simulink model "model_quad_linear_mpc_est"  (R2021b)
settings: Solver=FixedStepAuto  StartTime=0.0  StopTime=30  FixedStep=.025  RelTol=1e-3
values from neighbouring files (symbols this model uses):
  A = reshape([mt1,mt2,mt3,mt4,mt5,mt6,mt7,mt8],12,12)    [Jacob.m]    (also in Lineared_SS_model.m = reshape([-1.097500e-06;0.000000e+00;0.000000e+00;-4.432200e-; find_optimal_lqr.m = reshape([-1.097500e-06;0.000000e+00;0.000000e+00;-4.432200e-; start_drone.m = zeros(12))
  B = reshape([mt9,mt10],12,4)    [Jacob.m]    (also in Lineared_SS_model.m = reshape([0.000000e+00;0.000000e+00;0.000000e+00;0.000000e+00; find_optimal_lqr.m = reshape([0.000000e+00;0.000000e+00;0.000000e+00;0.000000e+00; nlStateFcn.m = [0 0 0]; start_drone.m = zeros(12,4))
libraries: mpclib x6
settings Model: Creator=Elena  LastModifiedBy=Elena

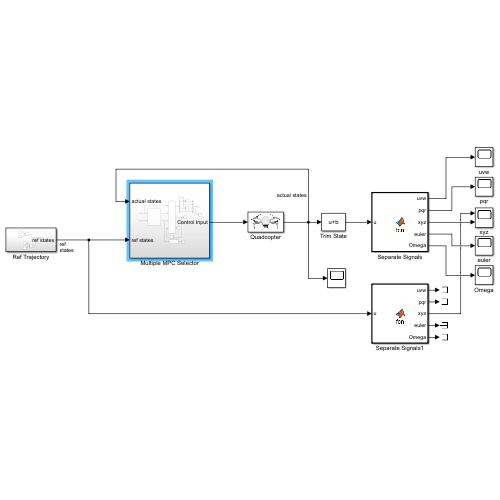
[thumbnail: Simulink's stored preview of the top-level diagram]
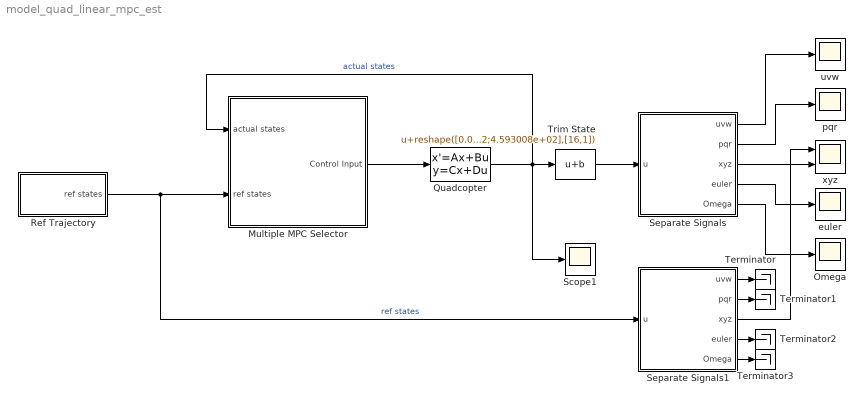
== system model_quad_linear_mpc_est ==
  Multiple MPC Selector : Subsystem
  Omega : Scope
  Quadcopter : StateSpace  A=A  B=B  C=eye(16)  D=zeros(16,4)  InitialCondition=0
      mask Display: image('drone_model.png'); % Use "Edit Image" on toolstrip to change.
  Ref Trajectory : Subsystem
  Scope1 : Scope
  Separate Signals : MATLAB Function  TreatAsAtomicUnit=on
  Separate Signals1 : MATLAB Function  TreatAsAtomicUnit=on
  Terminator{,1..3} (4 alike) : Terminator
  Trim State : Bias  Bias=reshape([0.000000e+00;0.000000e+00;0.000000e+00;0.000000e+00;0.000000e+00;0.000000e+00;0.000000e+00;0.000000e+00;0.000000e+00;0.000000e+00;0.000000e+00;0.000000e+00;0;4.593008e+02;4.593008e+02;4.593008e+02],[16,1])
  euler : Scope
  pqr : Scope
  uvw : Scope
  xyz : Scope  NumInputPorts=2
  wires:
  Quadcopter/1 -> Multiple MPC Selector/1(actual states), Trim State/1, Scope1/1  "actual states"
  Separate Signals/3(xyz) -> xyz/2
  Separate Signals/2(pqr) -> pqr/1
  Separate Signals/1(uvw) -> uvw/1
  Separate Signals/4(euler) -> euler/1
  Separate Signals/5(Omega) -> Omega/1
  Trim State/1 -> Separate Signals/1(u)
  Separate Signals1/3(xyz) -> xyz/1
  Separate Signals1/1(uvw) -> Terminator/1
  Separate Signals1/2(pqr) -> Terminator1/1
  Separate Signals1/4(euler) -> Terminator2/1
  Separate Signals1/5(Omega) -> Terminator3/1
  Ref Trajectory/1(ref states) -> Separate Signals1/1(u), Multiple MPC Selector/2(ref states)  "ref states"
  Multiple MPC Selector/1(Control Input) -> Quadcopter/1

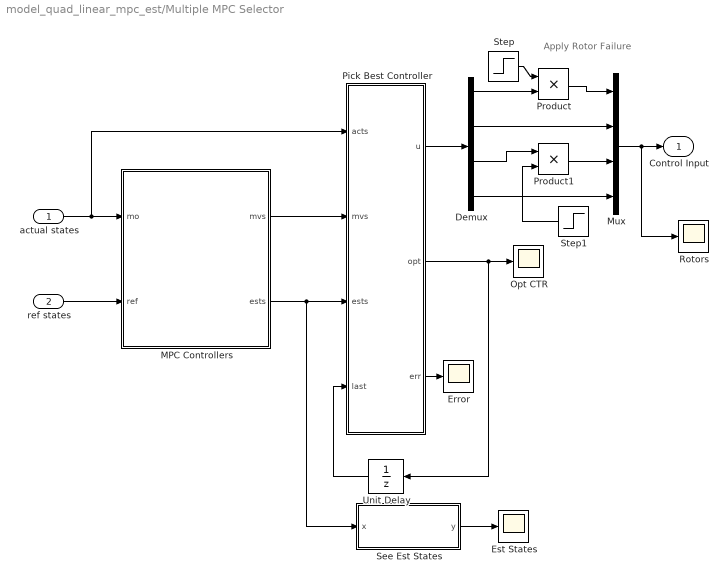
== system model_quad_linear_mpc_est/Multiple MPC Selector ==
  note: Apply Rotor Failure
  actual states : Inport
  ref states : Inport  Port=2
  Demux : Demux
  Error : Scope
  Est States : Scope
  MPC Controllers : Subsystem
  Mux : Mux
  Opt CTR : Scope
  Pick Best Controller : MATLAB Function  TreatAsAtomicUnit=on
  Product : Product
  Product1 : Product
  Rotors : Scope
  See Est States : MATLAB Function  TreatAsAtomicUnit=on
  Step : Step  Time=11  Before=1  After=0  SampleTime=0
  Step1 : Step  Time=21  Before=1  After=0  SampleTime=0
  Unit Delay : UnitDelay  SampleTime=-1  HasFrameUpgradeWarning=on
  Control Input : Outport
  wires:
  actual states/1 -> MPC Controllers/1(mo), Pick Best Controller/1(acts)
  Pick Best Controller/2(opt) -> Opt CTR/1, Unit Delay/1
  Pick Best Controller/3(err) -> Error/1
  Unit Delay/1 -> Pick Best Controller/4(last)
  ref states/1 -> MPC Controllers/2(ref)
  MPC Controllers/1(mvs) -> Pick Best Controller/2(mvs)
  MPC Controllers/2(ests) -> See Est States/1(x), Pick Best Controller/3(ests)
  Demux/2 -> Mux/2
  Step/1 -> Product/1
  Product/1 -> Mux/1
  Mux/1 -> Rotors/1, Control Input/1
  Demux/3 -> Product1/1
  Pick Best Controller/1(u) -> Demux/1
  Demux/1 -> Product/2
  Demux/4 -> Mux/4
  See Est States/1(y) -> Est States/1
  Product1/1 -> Mux/3
  Step1/1 -> Product1/2

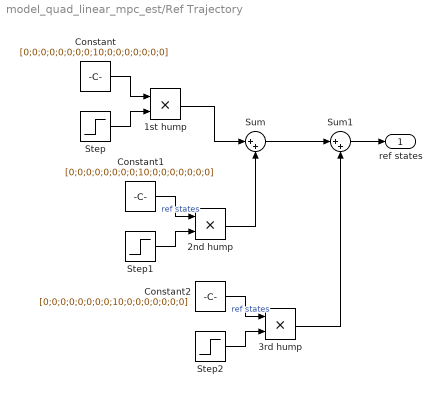
== system model_quad_linear_mpc_est/Ref Trajectory ==
  1st hump : Product
  2nd hump : Product
  3rd hump : Product
  Constant : Constant  Value=[0;0;0;0;0;0;0;0;10;0;0;0;0;0;0;0]
  Constant1 : Constant  Value=[0;0;0;0;0;0;0;0;10;0;0;0;0;0;0;0]
  Constant2 : Constant  Value=[0;0;0;0;0;0;0;0;10;0;0;0;0;0;0;0]
  Step : Step  SampleTime=0
  Step1 : Step  Time=10  SampleTime=0
  Step2 : Step  Time=20  SampleTime=0
  Sum : Sum  Inputs=|++
  Sum1 : Sum  Inputs=|++
  ref states : Outport
  wires:
  Step/1 -> 1st hump/2
  Constant/1 -> 1st hump/1
  Sum1/1 -> ref states/1
  2nd hump/1 -> Sum/2
  Constant1/1 -> 2nd hump/1  "ref states"
  Step1/1 -> 2nd hump/2
  1st hump/1 -> Sum/1
  Constant2/1 -> 3rd hump/1  "ref states"
  3rd hump/1 -> Sum1/2
  Step2/1 -> 3rd hump/2
  Sum/1 -> Sum1/1

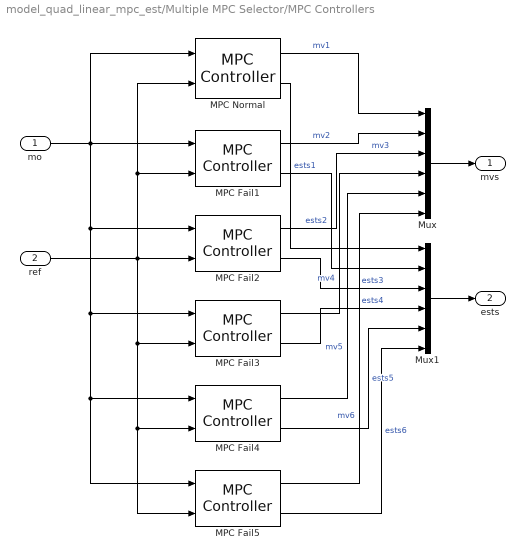
== system model_quad_linear_mpc_est/Multiple MPC Selector/MPC Controllers ==
  mo : Inport
  ref : Inport  Port=2
  MPC Fail1 : mpclib/MPC Controller  SCDEnableBlockLinearizationSpecification=on  mpcobj=mpc_l_fail_1  is_multiple=0  enable_value=0  return_u0=off  updateMPCinCallerWorkspace=on  md_inport=off  mv_inport=off  uref_inport=off  return_cost=off  return_mvseq=off  return_qpstatus=off  return_xseq=off  return_state=on  return_ovseq=off  state_inport=off  umin_inport=off  umax_inport=off  ymin_inport=off  ymax_inport=off  cc_inport=off  ywt_inport=off  uwt_inport=off  duwt_inport=off  rhoeps_inport=off  pm_inport=off  MaximumP=10  HorizonChoice=FixedHorizon  n_ts=0.1  n_p=20  n_mv=4  n_md=0  n_ud=0  n_mo=16  n_uo=0  BlockDataType=double  SampleTimeInherited=off  switch_inport=off
  MPC Fail2 : mpclib/MPC Controller  SCDEnableBlockLinearizationSpecification=on  mpcobj=mpc_l_fail_2  is_multiple=0  enable_value=0  return_u0=off  updateMPCinCallerWorkspace=on  md_inport=off  mv_inport=off  uref_inport=off  return_cost=off  return_mvseq=off  return_qpstatus=off  return_xseq=off  return_state=on  return_ovseq=off  state_inport=off  umin_inport=off  umax_inport=off  ymin_inport=off  ymax_inport=off  cc_inport=off  ywt_inport=off  uwt_inport=off  duwt_inport=off  rhoeps_inport=off  pm_inport=off  MaximumP=10  HorizonChoice=FixedHorizon  n_ts=0.1  n_p=20  n_mv=4  n_md=0  n_ud=0  n_mo=16  n_uo=0  BlockDataType=double  SampleTimeInherited=off  switch_inport=off
  MPC Fail3 : mpclib/MPC Controller  SCDEnableBlockLinearizationSpecification=on  mpcobj=mpc_l_fail_3  is_multiple=0  enable_value=0  return_u0=off  updateMPCinCallerWorkspace=on  md_inport=off  mv_inport=off  uref_inport=off  return_cost=off  return_mvseq=off  return_qpstatus=off  return_xseq=off  return_state=on  return_ovseq=off  state_inport=off  umin_inport=off  umax_inport=off  ymin_inport=off  ymax_inport=off  cc_inport=off  ywt_inport=off  uwt_inport=off  duwt_inport=off  rhoeps_inport=off  pm_inport=off  MaximumP=10  HorizonChoice=FixedHorizon  n_ts=0.1  n_p=20  n_mv=4  n_md=0  n_ud=0  n_mo=16  n_uo=0  BlockDataType=double  SampleTimeInherited=off  switch_inport=off
  MPC Fail4 : mpclib/MPC Controller  SCDEnableBlockLinearizationSpecification=on  mpcobj=mpc_l_fail_4  is_multiple=0  enable_value=0  return_u0=off  updateMPCinCallerWorkspace=on  md_inport=off  mv_inport=off  uref_inport=off  return_cost=off  return_mvseq=off  return_qpstatus=off  return_xseq=off  return_state=on  return_ovseq=off  state_inport=off  umin_inport=off  umax_inport=off  ymin_inport=off  ymax_inport=off  cc_inport=off  ywt_inport=off  uwt_inport=off  duwt_inport=off  rhoeps_inport=off  pm_inport=off  MaximumP=10  HorizonChoice=FixedHorizon  n_ts=0.1  n_p=20  n_mv=4  n_md=0  n_ud=0  n_mo=16  n_uo=0  BlockDataType=double  SampleTimeInherited=off  switch_inport=off
  MPC Fail5 : mpclib/MPC Controller  SCDEnableBlockLinearizationSpecification=on  mpcobj=mpc_l_fail_5  is_multiple=0  enable_value=0  return_u0=off  updateMPCinCallerWorkspace=on  md_inport=off  mv_inport=off  uref_inport=off  return_cost=off  return_mvseq=off  return_qpstatus=off  return_xseq=off  return_state=on  return_ovseq=off  state_inport=off  umin_inport=off  umax_inport=off  ymin_inport=off  ymax_inport=off  cc_inport=off  ywt_inport=off  uwt_inport=off  duwt_inport=off  rhoeps_inport=off  pm_inport=off  MaximumP=10  HorizonChoice=FixedHorizon  n_ts=0.1  n_p=20  n_mv=4  n_md=0  n_ud=0  n_mo=16  n_uo=0  BlockDataType=double  SampleTimeInherited=off  switch_inport=off
  MPC Normal : mpclib/MPC Controller  SCDEnableBlockLinearizationSpecification=on  mpcobj=mpc_l  is_multiple=0  enable_value=0  return_u0=off  updateMPCinCallerWorkspace=on  md_inport=off  mv_inport=off  uref_inport=off  return_cost=off  return_mvseq=off  return_qpstatus=off  return_xseq=off  return_state=on  return_ovseq=off  state_inport=off  umin_inport=off  umax_inport=off  ymin_inport=off  ymax_inport=off  cc_inport=off  ywt_inport=off  uwt_inport=off  duwt_inport=off  rhoeps_inport=off  pm_inport=off  MaximumP=10  HorizonChoice=FixedHorizon  n_ts=0.1  n_p=20  n_mv=4  n_md=0  n_ud=0  n_mo=16  n_uo=0  BlockDataType=double  SampleTimeInherited=off  switch_inport=off
  Mux : Mux  Inputs=6
  Mux1 : Mux  Inputs=6
  mvs : Outport
  ests : Outport  Port=2
  wires:
  ref/1 -> MPC Fail5/2, MPC Fail4/2, MPC Fail3/2, MPC Normal/2, MPC Fail1/2, MPC Fail2/2
  MPC Normal/2 -> Mux1/1  "ests1"
  MPC Fail4/1 -> Mux/5  "mv5"
  MPC Fail2/1 -> Mux/3  "mv3"
  MPC Fail3/1 -> Mux/4  "mv4"
  MPC Fail4/2 -> Mux1/5  "ests5"
  MPC Fail1/1 -> Mux/2  "mv2"
  Mux1/1 -> ests/1
  MPC Fail2/2 -> Mux1/3  "ests3"
  MPC Fail1/2 -> Mux1/2  "ests2"
  MPC Fail3/2 -> Mux1/4  "ests4"
  MPC Normal/1 -> Mux/1  "mv1"
  mo/1 -> MPC Normal/1, MPC Fail1/1, MPC Fail5/1, MPC Fail4/1, MPC Fail3/1, MPC Fail2/1
  Mux/1 -> mvs/1
  MPC Fail5/1 -> Mux/6  "mv6"
  MPC Fail5/2 -> Mux1/6  "ests6"

== matlab function model_quad_linear_mpc_est/Separate Signals1 ==
  data: u input; uvw output; pqr output; xyz output; euler output; Omega output
function [uvw,pqr,xyz,euler,Omega] = fcn(u)

uvw=u(1:3);
pqr=u((1:3)+3);
xyz=u((1:3)+6);
euler=u((1:3)+9);
Omega=u((1:4)+12);

== matlab function model_quad_linear_mpc_est/Separate Signals ==
  data: u input; uvw output; pqr output; xyz output; euler output; Omega output
function [uvw,pqr,xyz,euler,Omega] = fcn(u)

uvw=u(1:3);
pqr=u((1:3)+3);
xyz=u((1:3)+6);
euler=u((1:3)+9);
Omega=u((1:4)+12);

== matlab function model_quad_linear_mpc_est/Multiple MPC Selector/Pick Best Controller ==
  data: acts input; mvs input; u output; ests input; opt output; err output; last input
function [u,opt,err] = fcn(acts,mvs,ests,last)

% Set initial controller
if last == 0
    last = 1;
end

% This part assumes that if a fault has been detected, it will not be resolved
  

% For each controller compare XYZ actual states to ctr's est states
err = zeros(1,6);
for i = 0:5
    for ii = 7:9
        err(i+1) = err(i+1) + abs( acts(ii) - ests(ii+28*i) );
    end
end

[~,opt] = min(err); % Find most accurate controller

tol = .1;

if last == 1 % Controller hasn't changed
    if abs(err(last) - err(opt)) >= tol % Large difference in perf detected
        u = mvs(1+4*(opt-1):4+4*(opt-1)); % switch CTR
    else
        u = mvs(1+4*(last-1):4+4*(last-1)); % keep same CTR
        opt = last;
    end
else % Controller has previously changed
    if last >= 5 % Two rotors have failed
        u = mvs(1+4*(last-1):4+4*(last-1)); % keep same CTR
        opt = last;
    else % Only one rotor has failed
        if abs(err(last) - err(6)) >= tol % Large difference in perf detected (2nd rotor failed)
            u = mvs(1+4*(6-1):4+4*(6-1)); % switch to CTR 6
        else 
            u = mvs(1+4*(last-1):4+4*(last-1)); % keep same CTR
            opt = last;
        end
    end
end

%% PREVIOUS VERSIONS

% if last == 1 % Controller hasn't changed
%     if abs(err(last) - err(opt)) >= .3 % Large difference in perf detected
%         u = mvs(1+4*(opt-1):4+4*(opt-1)); % switch CTR
%     else
%         u = mvs(1+4*(last-1):4+4*(last-1)); % keep same CTR
%         opt = last;
%     end
% else % Controller has previously changed
%     if last >= 6 % Two rotors have failed
%         u = mvs(1+4*(last-1):4+4*(last-1)); % keep same CTR
%         opt = last;
%     else % Only one rotor has failed
%         if abs(err(last) - err(opt)) >= .3 % Large difference in perf detected (2nd rotor failed)
%             u = mvs(1+4*(opt-1):4+4*(opt-1)); % switch CTR
%         end
%     end
% end


% if big difference exists between current and optimal controller
% if abs(err(last) - err(opt)) >= .3
%     % switch controllers
%     u = mvs(1+4*(opt-1):4+4*(opt-1));
%     % else keep last one used
% else
%     u = mvs(1+4*(last-1):4+4*(last-1));
%     opt = last;
% end

end

== matlab function model_quad_linear_mpc_est/Multiple MPC Selector/See Est States ==
  data: x input; y output
function y = fcn(x)

y = zeros(1,length(x)/28);

for yy = 1:length(y)
    y(yy) = x(9+28*(yy-1));
end

end
